simulink model "SubSensor"  (R2020b)
settings: Solver=VariableStepAuto  StartTime=0.0  StopTime=10.0  RelTol=1e-3
settings Model: Creator=kaebi  LastModifiedBy=kaebi

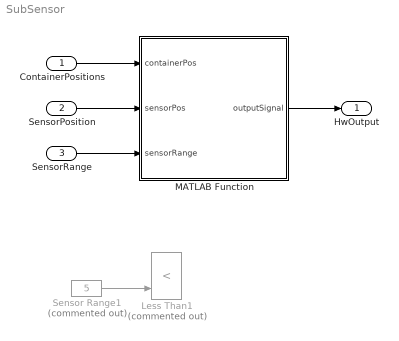
== system SubSensor ==
  ContainerPositions : Inport
  SensorPosition : Inport  Port=2
  SensorRange : Inport  Port=3
  Less Than1 : RelationalOperator  Commented=on  Operator=<  OutDataTypeStr=boolean  RndMeth=Simplest
  MATLAB Function : MATLAB Function  TreatAsAtomicUnit=on
  Sensor Range1 : Constant  Commented=on  Value=5
  HwOutput : Outport
  wires:
  SensorRange/1 -> MATLAB Function/3(sensorRange)
  ContainerPositions/1 -> MATLAB Function/1(containerPos)
  MATLAB Function/1(outputSignal) -> HwOutput/1
  SensorPosition/1 -> MATLAB Function/2(sensorPos)
  Sensor Range1/1 -> Less Than1/2

== matlab function SubSensor/MATLAB Function ==
  data: containerPos input; outputSignal output; sensorPos input; sensorRange input
function outputSignal = Sensor(containerPos, sensorPos, sensorRange)
    if (abs(sensorPos-containerPos) < sensorRange)
        outputSignal = 1;
    else
        outputSignal = 0;
    end
